simulink model "CTRL_LO_test"  (R2023b)
settings: Solver=VariableStepAuto  StartTime=0.0  StopTime=10.0  RelTol=1e-3
libraries: CTRL_LO x1, simulink x1
settings Model: Creator=blatak  LastModifiedBy=blatak

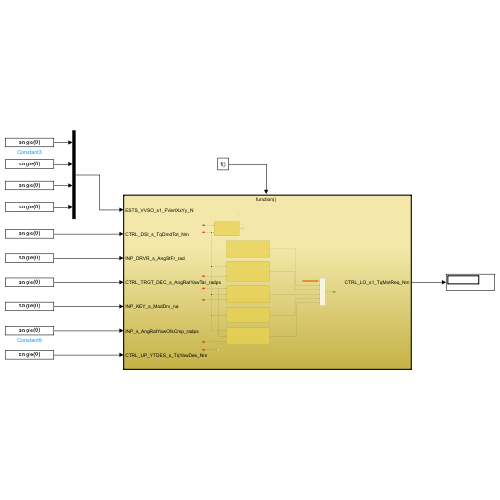
[thumbnail: Simulink's stored preview of the top-level diagram]
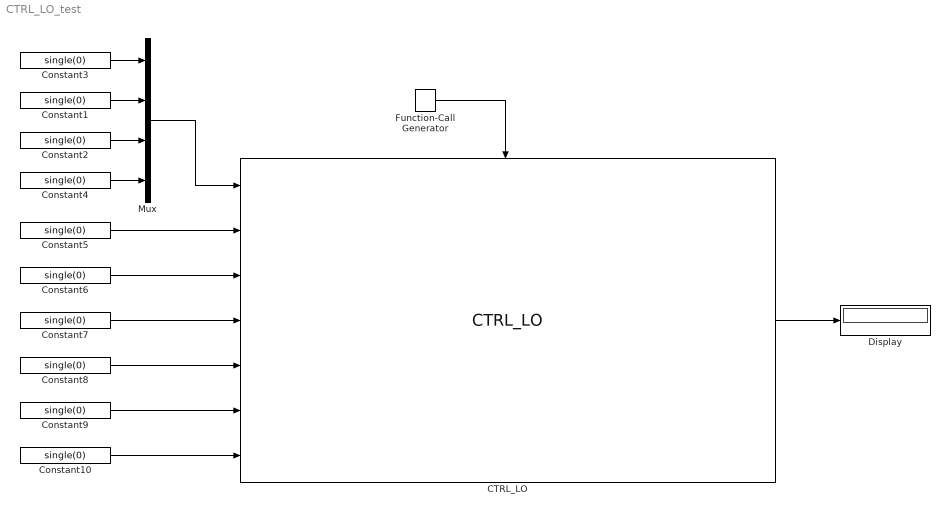
== system CTRL_LO_test ==
  CTRL_LO : CTRL_LO/CTRL_LO  SystemSampleTime=-1  VariantActivationTime=update diagram  AllowFlexibleInterface=on  Latency=0  AutoFrameSizeCalculation=off
  Constant{1..10} (10 alike) : Constant  Value=single(0)  OutDataTypeStr=single
  Display : Display
  Function-Call Generator : simulink/Ports & Subsystems/Function-Call Generator  sample_time=0.01  numberOfIterations=1  DisallowWideOutput=off
  Mux : Mux
  wires:
  Function-Call Generator/1 -> CTRL_LO/Trigger
  CTRL_LO/1 -> Display/1
  Constant9/1 -> CTRL_LO/6
  Constant8/1 -> CTRL_LO/5
  Constant7/1 -> CTRL_LO/4
  Constant6/1 -> CTRL_LO/3
  Constant5/1 -> CTRL_LO/2
  Constant4/1 -> Mux/4
  Constant2/1 -> Mux/3
  Constant1/1 -> Mux/2
  Constant3/1 -> Mux/1
  Mux/1 -> CTRL_LO/1
  Constant10/1 -> CTRL_LO/7
